simulink model "Day_Night_HLC"  (R2020a)
settings: Solver=FixedStepDiscrete  StartTime=0.0  StopTime=inf  FixedStep=1  RelTol=1e-3
undefined symbols (not defined in the file): DN, Ignition, Light, Road_T, sigbuilder_block
libraries: simulink x11
settings Model: Creator=VIJAY BANDEPPA MURGE  LastModifiedBy=VIJAY BANDEPPA MURGE

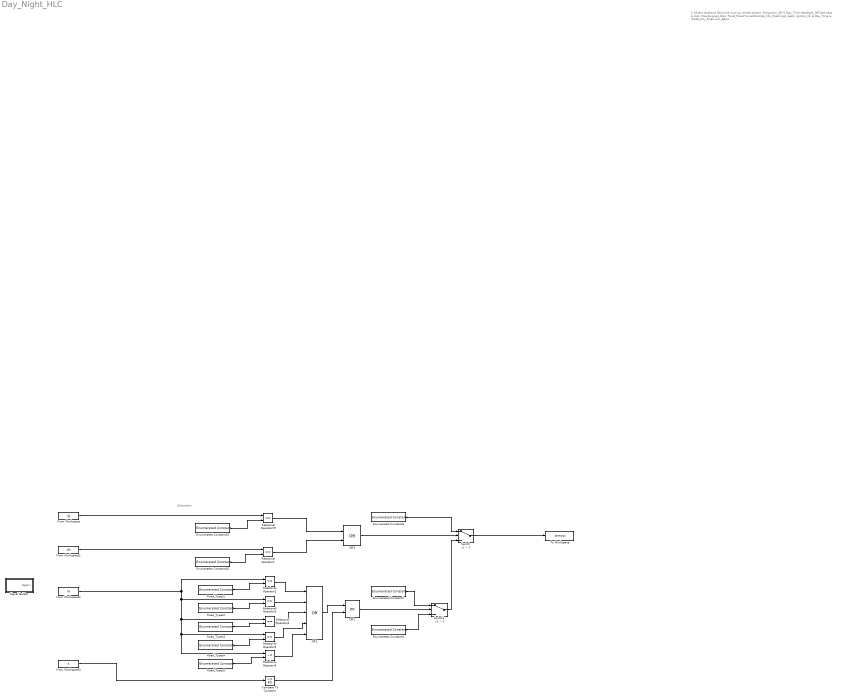
== system Day_Night_HLC ==
  note: Subsystem
  note: 1
      | Vikrant Gophane
      | Day-time running vehicle
      | Ignition_On/Ignition_Off & Day_Time
      | Headlight_Off
      |
      | Darkness & High_Way/Express_Way/ Rural_Road/Tunnel/Outside_City_Road
      | High_beam
      |
      | Ignition_On & Day_Time & InSide_City_Road
      | Low_Beam
  Compare To Constant : simulink/Logic and Bit Operations/Compare To Constant  relop=>=  const=60  OutDataTypeStr=boolean
  Enumerated Constant15 : simulink/Sources/Enumerated Constant  OutDataTypeStr=Enum: Ignition  Value=Ignition.Ignition_Off  SampleTime=inf
  Enumerated Constant16 : simulink/Sources/Enumerated Constant  OutDataTypeStr=Enum: DN  Value=DN.Day_Time  SampleTime=inf
  Enumerated Constant2 : simulink/Sources/Enumerated Constant  OutDataTypeStr=Enum: Light  Value=Light.High_beam  SampleTime=inf
  Enumerated Constant5 : simulink/Sources/Enumerated Constant  OutDataTypeStr=Enum: Light  Value=Light.Low_Beam  SampleTime=inf
  Enumerated Constant6 : simulink/Sources/Enumerated Constant  OutDataTypeStr=Enum: Light  Value=Light.Headlight_Off  SampleTime=inf
  From Workspace : FromWorkspace  VariableName=ig  OutDataTypeStr=Enum: Ignition
  From Workspace1 : FromWorkspace  VariableName=dn  OutDataTypeStr=Enum: DN
  From Workspace2 : FromWorkspace  VariableName=ro  OutDataTypeStr=Enum: Road_T
  From Workspace3 : FromWorkspace  VariableName=s
  OR1 : Logic  Operator=OR  Inputs=5  AllPortsSameDT=off  OutDataTypeStr=boolean
  OR2 : Logic  Operator=OR  AllPortsSameDT=off  OutDataTypeStr=boolean
  OR3 : Logic  Operator=OR  AllPortsSameDT=off  OutDataTypeStr=boolean
  Relational Operator{1..5,19} (6 alike) : RelationalOperator  Operator===  OutDataTypeStr=boolean  RndMeth=Simplest
  Relational Operator6 : RelationalOperator  Operator=~=  OutDataTypeStr=boolean  RndMeth=Simplest
  Road_Types1 : simulink/Sources/Enumerated Constant  OutDataTypeStr=Enum: Road_T  Value=Road_T.Express_Way  SampleTime=inf
  Road_Types2 : simulink/Sources/Enumerated Constant  OutDataTypeStr=Enum: Road_T  Value=Road_T.High_Way  SampleTime=inf
  Road_Types3 : simulink/Sources/Enumerated Constant  OutDataTypeStr=Enum: Road_T  Value=Road_T.Rural_Road  SampleTime=inf
  Road_Types4 : simulink/Sources/Enumerated Constant  OutDataTypeStr=Enum: Road_T  Value=Road_T.Outside_City_Road  SampleTime=inf
  Road_Types5 : simulink/Sources/Enumerated Constant  OutDataTypeStr=Enum: Road_T  Value=Road_T.Inside_City_Road  SampleTime=inf
  Signal Builder : Subsystem  Tag=STV Subsys  LoadFcn=sigbuilder_block('load',[437.6 199.2 550.4 400 ]);  StartFcn=sigbuilder_block('start');  StopFcn=sigbuilder_block('stop');  ClipboardFcn=sigbuilder_block('clipboard');  mask(Sigbuilder block){tuvar=[0:10]}
      mask help: Simulink:masks:SigbuilderBlock_MD
      mask init:
      | if ~strcmp(get_param(bdroot(gcbh),'SimulationStatus'),'stopped') tuvar = sigbuilder_block('maskInit'); end
      settings: CopyFcn=sigbuilder_block('copy');  DeleteFcn=sigbuilder_block('delete');  ModelCloseFcn=sigbuilder_block('modelClose');  PreSaveFcn=sigbuilder_block('preSave');  PauseFcn=sigbuilder_block('pause');  ContinueFcn=sigbuilder_block('continue');  NameChangeFcn=sigbuilder_block('namechange');  OpenFcn=sigbuilder_block('open',[437.6 199.2 550.4 400 ]);  CloseFcn=sigbuilder_block('close');
      mask Display: plot(0, 0, 100, 100,[2, 2, 32, 32, 2], [68, 8, 8, 68, 68],[32, 2], [38, 38], [32, 19, 2],[53, 60, 44], [32, 17, 17, 2],[16, 16, 31, 31]);txt = getActiveGroup(gcbh);text(2, 100, txt,'verticalAlignment', 'top');
  Switch : Switch  Criteria=u2 > Threshold
  Switch1 : Switch  Criteria=u2 > Threshold
  To Workspace : ToWorkspace  VariableName=simout  SaveFormat=Timeseries  SampleTime=-1
  wires:
  Switch/1 -> To Workspace/1
  Relational Operator5/1 -> OR1/4
  Relational Operator1/1 -> OR3/2
  Relational Operator3/1 -> OR1/2
  Relational Operator19/1 -> OR3/1
  From Workspace1/1 -> Relational Operator1/1
  Relational Operator4/1 -> OR1/3
  Switch1/1 -> Switch/3
  Enumerated Constant5/1 -> Switch1/3
  Road_Types3/1 -> Relational Operator4/2
  Enumerated Constant15/1 -> Relational Operator19/2
  Compare To Constant/1 -> OR2/2
  From Workspace2/1 -> Relational Operator6/1, Relational Operator5/1, Relational Operator4/1, Relational Operator3/1, Relational Operator2/1
  Relational Operator6/1 -> OR1/5
  OR3/1 -> Switch/2
  From Workspace3/1 -> Compare To Constant/1
  Enumerated Constant6/1 -> Switch/1
  Relational Operator2/1 -> OR1/1
  Enumerated Constant2/1 -> Switch1/1
  Enumerated Constant16/1 -> Relational Operator1/2
  OR2/1 -> Switch1/2
  Road_Types5/1 -> Relational Operator6/2
  OR1/1 -> OR2/1
  Road_Types4/1 -> Relational Operator5/2
  Road_Types1/1 -> Relational Operator2/2
  Road_Types2/1 -> Relational Operator3/2
  From Workspace/1 -> Relational Operator19/1

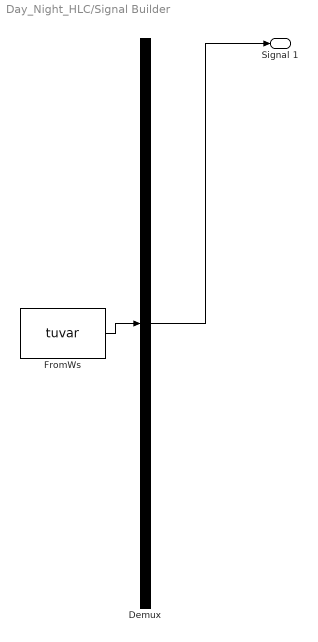
== system Day_Night_HLC/Signal Builder ==
  Demux : Demux  Tag=STV Demux  Outputs=1
      settings: DisplayOption=none
  FromWs : FromWorkspace  Tag=STV FromWs  VariableName=tuvar
      SigBuilderData=|
      | common.afterFinalStr = 'Extrapolate'
      | common.sampleTime = 0
      | dataSet.timeRange = [0 10]
      | dataSet.name = 'Group 1'
      | sbobj.Groups.Name = 'Group 1'
      | sbobj.Groups.Signals.Name = 'Signal 1'
      | sbobj.Groups.Signals.XData = [0 4 4 6 6 10]
      | sbobj.Groups.Signals.YData = [0 0 1 1 0 0]
  Signal 1 : Outport  Tag=STV Outport
  wires:
  Demux/1 -> Signal 1/1
  FromWs/1 -> Demux/1
